simulink model "friction_observer"  (R2021a)
settings: Solver=FixedStepAuto  StartTime=0.0  StopTime=10.0  RelTol=1e-3
model workspace (MAT data in the model file):
  C = [1  0  0  0  0  0  0  0; 0  1  0  0  0  0  0  0; 0  0  1  0  0  0  0  0; 0  0  0  1  0  0  0  0]
  Gamma = [0.005  0  0  0; 0  0.005  0  0; 0  0  0.005  0; 0  0  0  0.005; 0  0  0  0; 0  0  0  0; 0  0  0  0; 0  0  0  0]
  H = [-0.00548976801125  0  0  0; 0  -0.00548976801125  0  0; 0  0  -0.00778153069326  0; 0  0  0  -0.00778153069326; 7.42278491662  0  0  0; 0  7.42278491662  0  0; 0  0  10.7692000834  0; 0  0  0  10.7692000834]
  L = [0.929569914895  4.07390277635e-34  2.06829344266e-34  5.13045200608e-35; 7.44014379812e-35  0.929569914895  -3.30392036865e-18  1.96370039814e-17; -1.58638291611e-33  -2.78553325149e-17  0.929569914895  4.68164206202e-18; 1.63382777925e-34  -3.68097391751e-17  1.79546795367e-17  0.929569914895; -155.230736896  -2.03915068582e-31  -1.3281999231e-31  -1.68941834151e-32; -4.13497568008e-32  -155.230736896  1.72065563001e-15  -1.0226796559e-14; 8.36286019622e-31  1.48483522662e-14  -158.88512716  -2.49556060708e-15; -9.30261773711e-32  1.96215203609e-14  -9.57078528663e-15  -158.88512716]
  Li = [-1.1447690371  -6.16316458317e-33  -4.75950086043e-33  -2.75905944898e-34; -1.06322774158e-33  -1.1447690371  5.23444260855e-17  -3.11111524721e-16; 1.70837028089e-32  3.11342333157e-16  -0.80761956585  -5.23272648717e-17; -2.06171277528e-33  4.11426791318e-16  -2.00681568423e-16  -0.80761956585]
  M = 740
  Phi = [1  0  0  0  -0.00147916666667  0  0  0; 0  1  0  0  0  -0.00147916666667  0  0; 0  0  1  0  0  0  -0.00144514553226  0; 0  0  0  1  0  0  0  -0.00144514553226; 0  0  0  0  1  0  0  0; 0  0  0  0  0  1  0  0; 0  0  0  0  0  0  1  0; 0  0  0  0  0  0  0  1]
  Ts = 0.005
  g = 9.807
  h = 0.577
  l = 1.917
  lf = 1.036
  lr = 0.881
  re = 0.284
values from neighbouring files (symbols this model uses):
  Af = 1.6    [kf_dict.sldd]
  Cd = 0.3    [kf_dict.sldd]
  rho_air = 1.206    [kf_dict.sldd]
settings Model: DataDictionary=kf_dict.sldd  OrderedModelArguments=off  Creator=Henrique Mesquita  LastModifiedBy=Henrique Mesquita

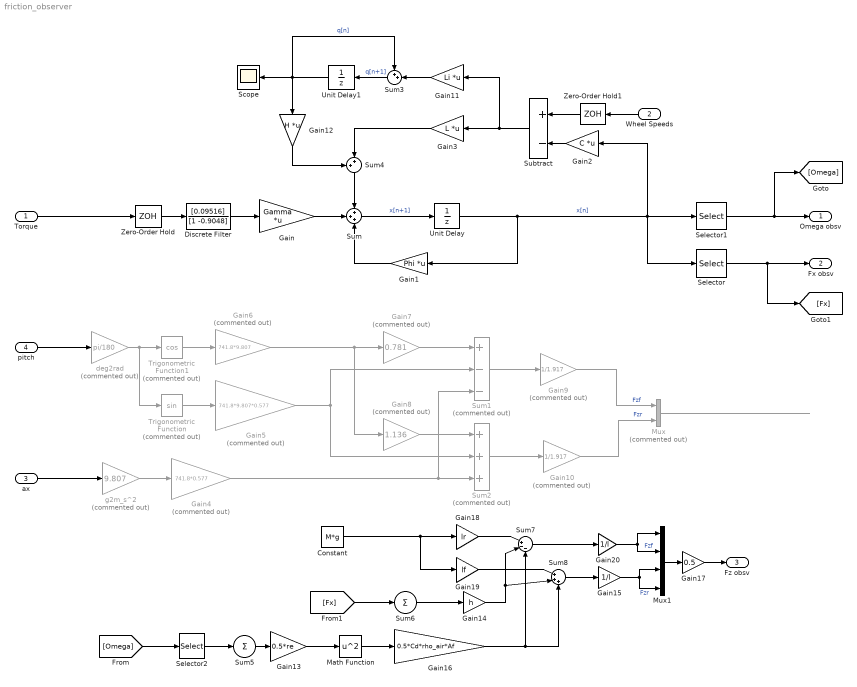
== system friction_observer ==
  Torque : Inport  PortDimensions=4
  Wheel Speeds : Inport  Port=2  PortDimensions=4
  ax : Inport  Port=3
  pitch : Inport  Port=4
  Constant : Constant  Value=M*g
  Discrete Filter : DiscreteFilter  Numerator=[0.09516]  Denominator=[1 -0.9048]
  Gain : Gain  Gain=Gamma  Multiplication=Matrix(K*u)
  Gain1 : Gain  Gain=Phi  Multiplication=Matrix(K*u)
  Gain10 : Gain  Commented=on  Gain=1/1.917
  Gain11 : Gain  Gain=Li  Multiplication=Matrix(K*u)
  Gain12 : Gain  Gain=H  Multiplication=Matrix(K*u)
  Gain13 : Gain  Gain=0.5*re
  Gain14 : Gain  Gain=h
  Gain15 : Gain  Gain=1/l
  Gain16 : Gain  Gain=0.5*Cd*rho_air*Af
  Gain17 : Gain  Gain=0.5
  Gain18 : Gain  Gain=lr
  Gain19 : Gain  Gain=lf
  Gain2 : Gain  Gain=C  Multiplication=Matrix(K*u)
  Gain20 : Gain  Gain=1/l
  Gain3 : Gain  Gain=L  Multiplication=Matrix(K*u)
  Gain4 : Gain  Commented=on  Gain=741.8*0.577
  Gain5 : Gain  Commented=on  Gain=741.8*9.807*0.577
  Gain6 : Gain  Commented=on  Gain=741.8*9.807
  Gain7 : Gain  Commented=on  Gain=0.781
  Gain8 : Gain  Commented=on  Gain=1.136
  Gain9 : Gain  Commented=on  Gain=1/1.917
  Math Function : Math  Operator=square  SaturateOnIntegerOverflow=on
  Mux : Mux  Commented=on  Inputs=2
  Mux1 : Mux
  Scope : Scope
  Selector : Selector  InputPortWidth=8  IndexOptions=Index vector (dialog)  Indices=[5 6 7 8]  OutputSizes=1
  Selector1 : Selector  InputPortWidth=8  IndexOptions=Index vector (dialog)  Indices=[1 2 3 4]  OutputSizes=1
  Selector2 : Selector  InputPortWidth=4  IndexOptions=Index vector (dialog)  Indices=[1 2]  OutputSizes=1
  Subtract : Sum  Inputs=+-
  Sum : Sum  Inputs=+++
  Sum1 : Sum  Commented=on  Inputs=+--
  Sum2 : Sum  Commented=on  Inputs=+++
  Sum3 : Sum  Inputs=++|
  Sum4 : Sum  Inputs=++|
  Sum5 : Sum  Inputs=+
  Sum6 : Sum  Inputs=+
  Sum7 : Sum  Inputs=|+--
  Sum8 : Sum  Inputs=|+++
  Trigonometric Function : Trigonometry  Commented=on
  Trigonometric Function1 : Trigonometry  Commented=on  Operator=cos
  Unit Delay : UnitDelay  SampleTime=Ts  HasFrameUpgradeWarning=on
  Unit Delay1 : UnitDelay  SampleTime=Ts  HasFrameUpgradeWarning=on
  Zero-Order Hold : ZeroOrderHold  SampleTime=Ts
  Zero-Order Hold1 : ZeroOrderHold  SampleTime=Ts
  deg2rad : Gain  Commented=on  Gain=pi/180
  g2m_s^2 : Gain  Commented=on  Gain=9.807
  Omega obsv : Outport
  Fx obsv : Outport  Port=2
  Fz obsv : Outport  Port=3
  wires:
  Torque/1 -> Zero-Order Hold/1
  Gain/1 -> Sum/2
  Sum/1 -> Unit Delay/1  "x[n+1]"
  Gain1/1 -> Sum/3
  Unit Delay/1 -> Selector1/1, Selector/1, Gain2/1, Gain1/1  "x[n]"
  Gain2/1 -> Subtract/2
  Wheel Speeds/1 -> Zero-Order Hold1/1
  Zero-Order Hold1/1 -> Subtract/1
  Selector1/1 -> [Omega], Omega obsv/1
  Selector/1 -> [Fx], Fx obsv/1
  Zero-Order Hold/1 -> Discrete Filter/1
  Discrete Filter/1 -> Gain/1
  pitch/1 -> deg2rad/1
  Trigonometric Function/1 -> Gain5/1
  Trigonometric Function1/1 -> Gain6/1
  Gain6/1 -> Gain8/1, Gain7/1
  Gain7/1 -> Sum1/1
  Gain8/1 -> Sum2/1
  Gain5/1 -> Sum2/2, Sum1/2
  ax/1 -> g2m_s^2/1
  Gain4/1 -> Sum1/3, Sum2/3
  Sum1/1 -> Gain9/1
  Sum2/1 -> Gain10/1
  Gain9/1 -> Mux/1  "Fzf"
  Gain10/1 -> Mux/2  "Fzr"
  Mux/1 -> ?
  Sum3/1 -> Unit Delay1/1  "q[n+1]"
  Gain11/1 -> Sum3/2
  Unit Delay1/1 -> Scope/1, Sum3/1, Gain12/1  "q[n]"
  Subtract/1 -> Gain3/1, Gain11/1
  Sum4/1 -> Sum/1
  Gain3/1 -> Sum4/2
  Gain12/1 -> Sum4/1
  deg2rad/1 -> Trigonometric Function/1, Trigonometric Function1/1
  g2m_s^2/1 -> Gain4/1
  Gain16/1 -> Sum8/3, Sum7/3
  Gain17/1 -> Fz obsv/1
  Mux1/1 -> Gain17/1
  [Fx] -> Sum6/1
  Constant/1 -> Gain19/1, Gain18/1
  Gain13/1 -> Math Function/1
  Gain18/1 -> Sum7/1
  [Omega] -> Selector2/1
  Sum6/1 -> Gain14/1
  Gain14/1 -> Sum8/2, Sum7/2
  Gain19/1 -> Sum8/1
  Gain15/1 -> Mux1/4, Mux1/3  "Fzr"
  Math Function/1 -> Gain16/1
  Gain20/1 -> Mux1/2, Mux1/1  "Fzf"
  Sum5/1 -> Gain13/1
  Sum7/1 -> Gain20/1
  Selector2/1 -> Sum5/1
  Sum8/1 -> Gain15/1
